simulink model "servomotor_posicao"  (R2019b)
settings: Solver=FixedStepAuto  StartTime=0.0  StopTime=tf  FixedStep=1e-6  RelTol=1e-3
values from neighbouring files (symbols this model uses):
  controlador =     [controlador.mat]    (also in projetarControladorCorrenteOtimizacao.m = projetarControladorCorrenteAnalitico(      requisitos, plant; projetarControladorPosicaoOtimizacao.m = projetarControladorPosicaoAnalitico(requisitos, planta))
  planta =     [controlador.mat]
settings Model: Creator=mmaximo  LastModifiedBy=freit

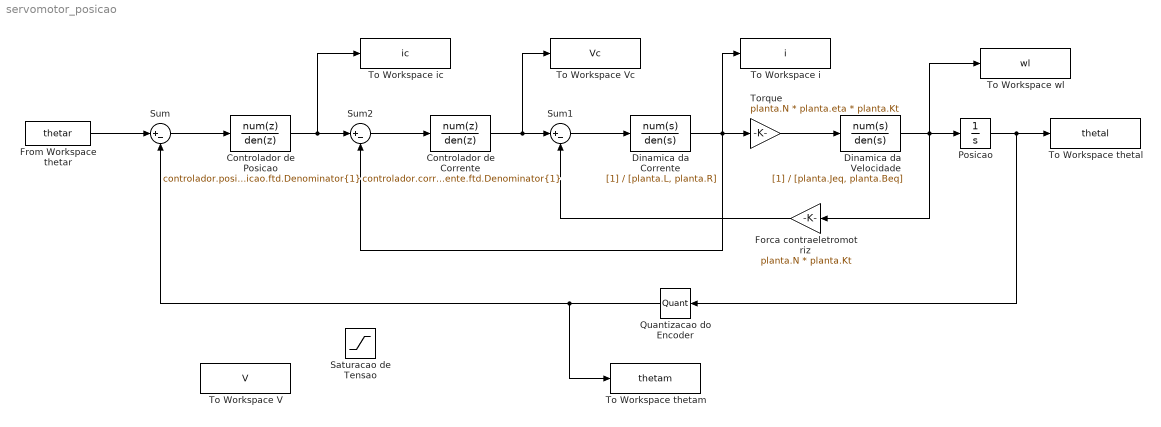
== system servomotor_posicao ==
  Controlador de Corrente : DiscreteTransferFcn  Numerator=controlador.corrente.ftd.Numerator{1}  Denominator=controlador.corrente.ftd.Denominator{1}  SampleTime=controlador.corrente.T
  Controlador de Posicao : DiscreteTransferFcn  Numerator=controlador.posicao.ftd.Numerator{1}  Denominator=controlador.posicao.ftd.Denominator{1}  SampleTime=controlador.posicao.T
  Dinamica da Corrente : TransferFcn  Denominator=[planta.L, planta.R]
  Dinamica da Velocidade : TransferFcn  Denominator=[planta.Jeq, planta.Beq]
  Forca contraeletromotriz : Gain  Gain=planta.N * planta.Kt
  From Workspace thetar : FromWorkspace  VariableName=thetar  SampleTime=0
  Posicao : Integrator
  Quantizacao do Encoder : Quantizer  QuantizationInterval=planta.quantizacaoEncoder
  Saturacao de Tensao : Saturate  UpperLimit=planta.Vmax  LowerLimit=-planta.Vmax
  Sum : Sum  Inputs=|+-
  Sum1 : Sum  Inputs=|+-
  Sum2 : Sum  Inputs=|+-
  To Workspace V : ToWorkspace  VariableName=V  SaveFormat=Structure With Time  SampleTime=1e-6
  To Workspace Vc : ToWorkspace  VariableName=Vc  SaveFormat=Structure With Time  SampleTime=1e-6
  To Workspace i : ToWorkspace  VariableName=i  SaveFormat=Structure With Time  SampleTime=1e-6
  To Workspace ic : ToWorkspace  VariableName=ic  SaveFormat=Structure With Time  SampleTime=1e-6
  To Workspace thetal : ToWorkspace  VariableName=thetal  SaveFormat=Structure With Time  SampleTime=-1
  To Workspace thetam : ToWorkspace  VariableName=thetam  SaveFormat=Structure With Time  SampleTime=-1
  To Workspace wl : ToWorkspace  VariableName=wl  SaveFormat=Structure With Time  SampleTime=1e-6
  Torque : Gain  Gain=planta.N * planta.eta * planta.Kt
  wires:
  From Workspace thetar/1 -> Sum/1
  Sum/1 -> Controlador de Posicao/1
  Controlador de Posicao/1 -> To Workspace ic/1, Sum2/1
  Sum2/1 -> Controlador de Corrente/1
  Controlador de Corrente/1 -> To Workspace Vc/1, Sum1/1
  Sum1/1 -> Dinamica da Corrente/1
  Torque/1 -> Dinamica da Velocidade/1
  Posicao/1 -> Quantizacao do Encoder/1, To Workspace thetal/1
  Dinamica da Corrente/1 -> To Workspace i/1, Sum2/2, Torque/1
  Dinamica da Velocidade/1 -> To Workspace wl/1, Forca contraeletromotriz/1, Posicao/1
  Forca contraeletromotriz/1 -> Sum1/2
  Quantizacao do Encoder/1 -> To Workspace thetam/1, Sum/2
